simulink model "motor_and_rod_model_simulink"  (R2023b)
settings: Solver=VariableStepAuto  StartTime=0.0  StopTime=50  RelTol=1e-3
values from neighbouring files (symbols this model uses):
  Br = 2.5592e-5    (= 2.5592e-05)    [DC_motor_and_Rod.m]
  Jm = 4e-6    (= 4e-06)    [DC_motor_and_Rod.m]
  Jr = 9.5958e-5    (= 9.5958e-05)    [DC_motor_and_Rod.m]
  Kc = 0.042    [DC_motor_and_Rod.m]
  Ke = 0.042    [DC_motor_and_Rod.m]
  omega0 = omega_vector(1)    [DC_motor_and_Rod.m]
  Ra = 8.4    [DC_motor_and_Rod.m]
settings Model: Creator=renzo  LastModifiedBy=renzo

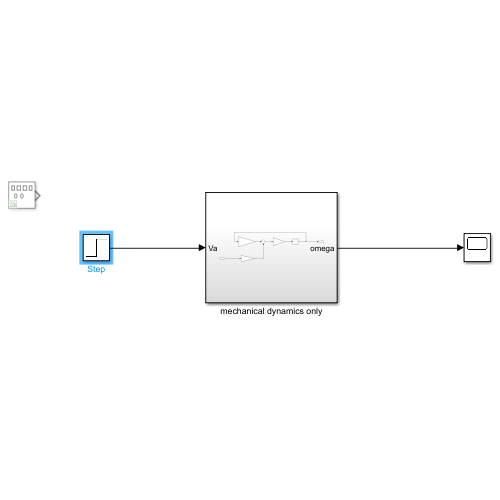
[thumbnail: Simulink's stored preview of the top-level diagram]
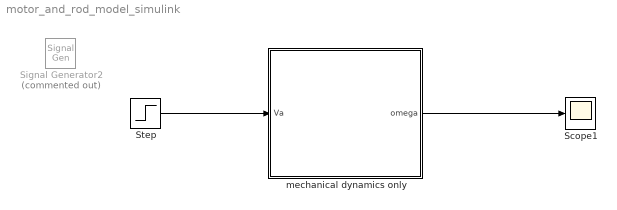
== system motor_and_rod_model_simulink ==
  Scope1 : Scope
  Signal Generator2 : SignalGenerator  Commented=on  WaveForm=square  Frequency=0.1
  Step : Step  Time=0  SampleTime=0
  mechanical dynamics only : Subsystem
  wires:
  mechanical dynamics only/1(omega) -> Scope1/1
  Step/1 -> mechanical dynamics only/1(Va)

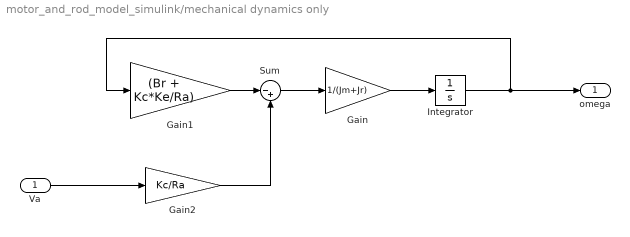
== system motor_and_rod_model_simulink/mechanical dynamics only ==
  Va : Inport
  Gain : Gain  Gain=1/(Jm+Jr)
  Gain1 : Gain  Gain=(Br + Kc*Ke/Ra)
  Gain2 : Gain  Gain=Kc/Ra
  Integrator : Integrator  InitialCondition=omega0
  Sum : Sum  Inputs=|-+
  omega : Outport
  wires:
  Sum/1 -> Gain/1
  Integrator/1 -> omega/1, Gain1/1
  Gain1/1 -> Sum/1
  Gain2/1 -> Sum/2
  Va/1 -> Gain2/1
  Gain/1 -> Integrator/1
